simulink model "simulation"  (R2023b)
settings: Solver=VariableStepAuto  StartTime=0.0  StopTime=12  RelTol=1e-5
values from neighbouring files (symbols this model uses):
  K_e = 10    [elastic_actuator.m]
libraries: cstblocks x2
settings Model: Creator=frenci  LastModifiedBy=frenci

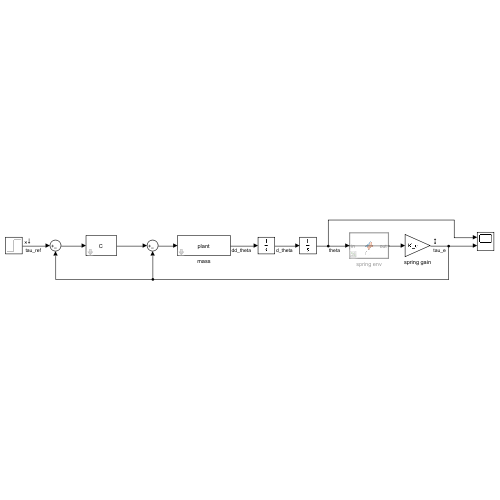
[thumbnail: Simulink's stored preview of the top-level diagram]
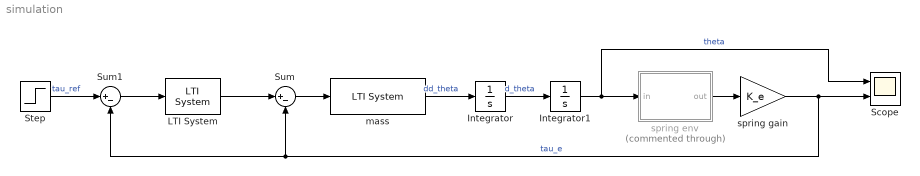
== system simulation ==
  Integrator : Integrator
  Integrator1 : Integrator
  LTI System : cstblocks/LTI System  sys=C  IC=[]  PadeOrder=0
  Scope : Scope  NumInputPorts=2
  Step : Step  SampleTime=0  VectorParams1D=off
  Sum : Sum  Inputs=|+-
  Sum1 : Sum  Inputs=|+-
  mass : cstblocks/LTI System  sys=plant  IC=[]  PadeOrder=0
  spring env : MATLAB Function  Commented=through  TreatAsAtomicUnit=on
  spring gain : Gain  Gain=K_e
  wires:
  Integrator/1 -> Integrator1/1  "d_theta"
  mass/1 -> Integrator/1  "dd_theta"
  Integrator1/1 -> Scope/1, spring env/1(in)  "theta"
  Sum/1 -> mass/1
  spring env/1(out) -> spring gain/1
  spring gain/1 -> Scope/2, Sum1/2, Sum/2  "tau_e"
  LTI System/1 -> Sum/1
  Step/1 -> Sum1/1  "tau_ref"
  Sum1/1 -> LTI System/1

== matlab function simulation/spring env ==
  data: in input; out output
function out = fcn(in)

theta_o=2;
distance=in(1)-theta_o;

if distance > 0
    force= distance;
else
    force=0;

end


out = force;
